simulink model "ProjectEdge"  (R2020a)
settings: Solver=VariableStepAuto  StartTime=0.0  StopTime=10  RelTol=1e-3
settings Model: Creator=mario  LastModifiedBy=mario

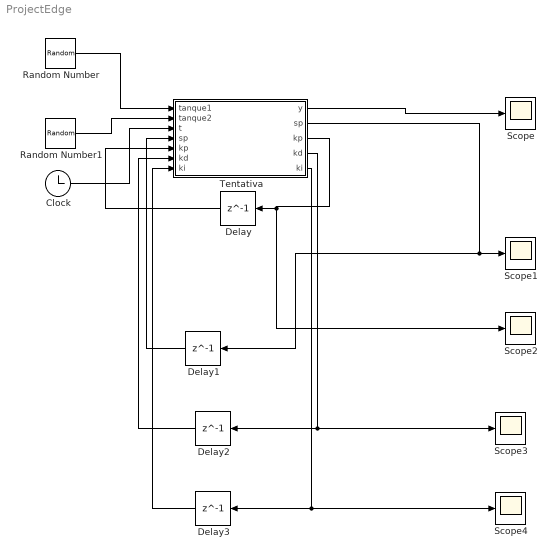
== system ProjectEdge ==
  Clock : Clock
  Delay{,1..3} (4 alike) : Delay  DelayLength=1  InitialCondition=0
  Random Number : RandomNumber  SampleTime=0.1
  Random Number1 : RandomNumber  SampleTime=0.1
  Scope{,1..4} (5 alike) : Scope
  Tentativa : MATLAB Function  TreatAsAtomicUnit=on
  wires:
  Random Number/1 -> Tentativa/1(tanque1)
  Tentativa/1(y) -> Scope/1
  Clock/1 -> Tentativa/3(t)
  Delay/1 -> Tentativa/5("kp ")
  Tentativa/3(kp) -> Scope2/1, Delay/1
  Tentativa/2(sp) -> Delay1/1, Scope1/1
  Delay1/1 -> Tentativa/4("sp ")
  Random Number1/1 -> Tentativa/2(tanque2)
  Tentativa/4(kd) -> Scope3/1, Delay2/1
  Tentativa/5(ki) -> Scope4/1, Delay3/1
  Delay3/1 -> Tentativa/7("ki ")
  Delay2/1 -> Tentativa/6("kd ")

== matlab function ProjectEdge/Tentativa ==
  data: tanque1 input; tanque2 input; y output; t input; sp output; kp output; sp input; kp input; kd input; ki input; kd output; ki output
function [y,sp,kp, kd, ki]   = Conexao1(tanque1,tanque2,t,sp, kp, kd, ki)
y = 0;
sp  = sp;
kp = kp; 
kd = kd;
ki = ki;
coder.extrinsic('py.T3.conexao');
if(mod(t,.2) == 0)
   msg = char(py.T3.conexao(sprintf("%.4f",tanque1),sprintf("%.4f",tanque2)));
   disp(msg)
   sp = str2double(msg(6:13));
   kp = str2double(msg(18:25));
   kd = str2double(msg(30:37));
   ki = str2double(msg((42:49)));  
end
end
